simulink model "gm_ZedBoardTest"  (R2014b)
settings: Solver=FixedStepDiscrete  SolverMode=SingleTasking  StartTime=0.0  StopTime=10  RelTol=1e-3
InitFcn:
  | Ts = 1e-3;
settings Model: Creator=wchen  LastModifiedBy=dlwalter
settings DataIOCC: SaveOutput=off  SignalLogging=off  SaveTime=off
settings OptimizationCC: BlockReduction=off  ConditionallyExecuteInputs=off  InlineParams=on  ExpressionDepthLimit=2147483647
settings DebuggingCC: AlgebraicLoopMsg=error  UnderspecifiedInitializationDetection=Classic  MergeDetectMultiDrivingBlocksExec=none  InheritedTsInSrcMsg=none  SingleTaskRateTransMsg=error  ParameterPrecisionLossMsg=none  StateNameClashWarn=warning
settings HardwareCC: ProdHWDeviceType=ASIC/FPGA->ASIC/FPGA  ProdEqTarget=off

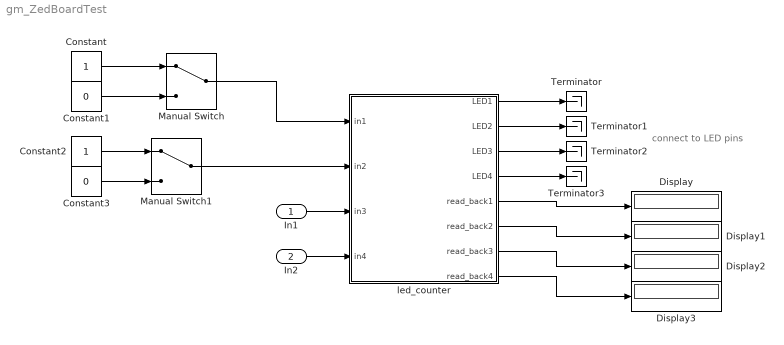
== system gm_ZedBoardTest ==
  note: connect to
      | LED pins
  In1 : Inport
  In2 : Inport  Port=2
  Constant : Constant  OutDataTypeStr=boolean  SampleTime=Ts
  Constant1 : Constant  Value=0  OutDataTypeStr=boolean  SampleTime=Ts
  Constant2 : Constant  OutDataTypeStr=boolean  SampleTime=Ts
  Constant3 : Constant  Value=0  OutDataTypeStr=boolean  SampleTime=Ts
  Display{,1..3} (4 alike) : Display
  Manual Switch : ManualSwitch
  Manual Switch1 : ManualSwitch
  Terminator{,1..3} (4 alike) : Terminator
  led_counter : Subsystem  TreatAsAtomicUnit=on
  wires:
  In2/1 -> led_counter/4(in4)
  In1/1 -> led_counter/3(in3)
  led_counter/8(read_back4) -> Display3/1
  led_counter/7(read_back3) -> Display2/1
  led_counter/6(read_back2) -> Display1/1
  led_counter/5(read_back1) -> Display/1
  led_counter/4(LED4) -> Terminator3/1
  led_counter/3(LED3) -> Terminator2/1
  led_counter/2(LED2) -> Terminator1/1
  led_counter/1(LED1) -> Terminator/1
  Manual Switch1/1 -> led_counter/2(in2)
  Constant3/1 -> Manual Switch1/2
  Constant2/1 -> Manual Switch1/1
  Manual Switch/1 -> led_counter/1(in1)
  Constant1/1 -> Manual Switch/2
  Constant/1 -> Manual Switch/1

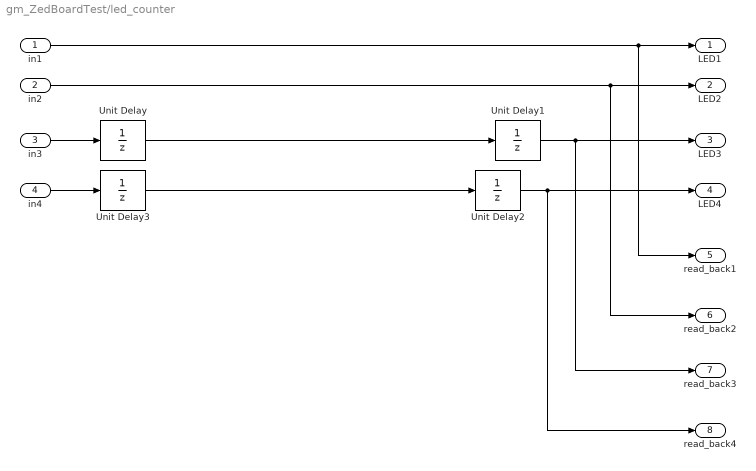
== system gm_ZedBoardTest/led_counter ==
  in1 : Inport  OutDataTypeStr=boolean
  in2 : Inport  Port=2  OutDataTypeStr=boolean
  in3 : Inport  Port=3  OutDataTypeStr=boolean
  in4 : Inport  Port=4  OutDataTypeStr=boolean
  Unit Delay{,1..3} (4 alike) : UnitDelay  SampleTime=-1
  LED1 : Outport
  LED2 : Outport  Port=2
  LED3 : Outport  Port=3
  LED4 : Outport  Port=4
  read_back1 : Outport  Port=5
  read_back2 : Outport  Port=6
  read_back3 : Outport  Port=7
  read_back4 : Outport  Port=8
  wires:
  Unit Delay3/1 -> Unit Delay2/1
  Unit Delay2/1 -> LED4/1, read_back4/1
  Unit Delay1/1 -> LED3/1, read_back3/1
  Unit Delay/1 -> Unit Delay1/1
  in4/1 -> Unit Delay3/1
  in3/1 -> Unit Delay/1
  in2/1 -> LED2/1, read_back2/1
  in1/1 -> LED1/1, read_back1/1
